simulink model "Tire_Presssure_Lamp_Model"  (R2024a)
settings: Solver=VariableStepAuto  StartTime=0.0  StopTime=10  RelTol=1e-3
settings Model: Creator=ec97883  LastModifiedBy=ec97883

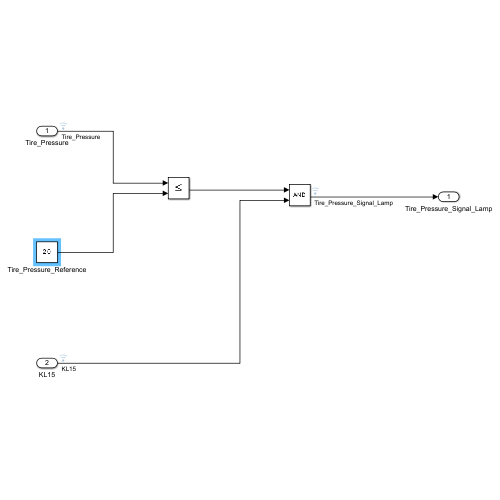
[thumbnail: Simulink's stored preview of the top-level diagram]
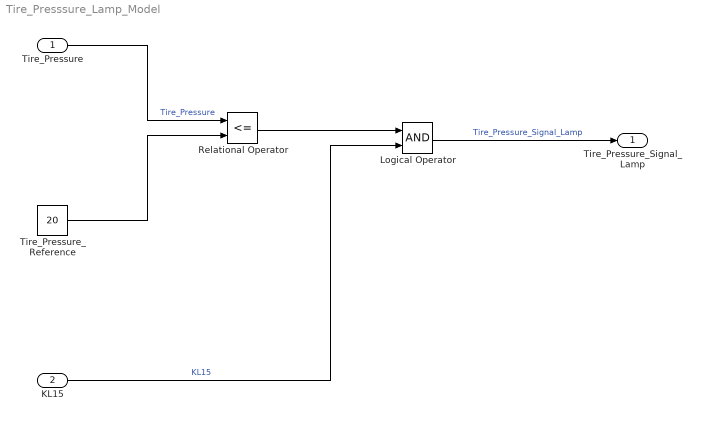
== system Tire_Presssure_Lamp_Model ==
  Tire_Pressure : Inport  OutDataTypeStr=uint32
  KL15 : Inport  Port=2  OutDataTypeStr=boolean  PortDimensions=1
  Logical Operator : Logic  AllPortsSameDT=off  OutDataTypeStr=boolean
  Relational Operator : RelationalOperator  Operator=<=  OutDataTypeStr=boolean  RndMeth=Simplest  InputSameDT=off
  Tire_Pressure_Reference : Constant  Value=20  OutDataTypeStr=uint32
  Tire_Pressure_Signal_Lamp : Outport  OutDataTypeStr=boolean  PortDimensions=1
  wires:
  Tire_Pressure/1 -> Relational Operator/1  "Tire_Pressure"
  Tire_Pressure_Reference/1 -> Relational Operator/2
  Relational Operator/1 -> Logical Operator/1
  KL15/1 -> Logical Operator/2  "KL15"
  Logical Operator/1 -> Tire_Pressure_Signal_Lamp/1  "Tire_Pressure_Signal_Lamp"
